simulink model "CACC_4_Robots"  (R2021a)
settings: Solver=FixedStepAuto  StartTime=0.0  StopTime=Tsim  RelTol=1e-3
values from neighbouring files (symbols this model uses):
  h = 1.0    (= 1)    [ros_cacc.m]    (also in ros_cacc2.m)
  k1 = 1    [ros_cacc.m]    (also in ros_cacc2.m)
  k2 = 1    [ros_cacc.m]    (also in ros_cacc2.m)
  r = 1    [ros_cacc.m]    (also in ros_cacc2.m)
  v_0 = 0.5    [ros_cacc.m]    (also in ros_cacc2.m)
  v_threshold = v_thr    (= 0.1)    [ros_cacc.m]    (also in ros_cacc2.m)
undefined symbols (not defined in the file or in its folder): angular, linear
libraries: ros2lib x17, robotcorelib x4
(part 3 of 3)

== system CACC_4_Robots/Subsystem2/controllers/Switch Case Ext. LA/s/Approximation of s around zero ==
  In1 : Inport
  Action Port : ActionPort  ActionPortLabel=if(u1 < 0.01 & u1 > -0.01)
  Taylor approximation 3rd order : Fcn  Expr=0.5*(r+h*u(2))^2*u(1)-0.125*(r+h*u(2))^4*u(1)^3
  Out1 : Outport  VectorParamsAs1DForOutWhenUnconnected=off
  wires:
  In1/1 -> Taylor approximation 3rd order/1
  Taylor approximation 3rd order/1 -> Out1/1

== system CACC_4_Robots/Subsystem2/controllers/Switch Case Ext. LA/s/function s ==
  In1 : Inport
  Action Port : ActionPort  ActionPortLabel=else
  function s : Fcn  Expr=(-1+sqrt(1+u(1)^2*(r+h*u(2))^2))/u(1)
  Out1 : Outport  VectorParamsAs1DForOutWhenUnconnected=off
  wires:
  In1/1 -> function s/1
  function s/1 -> Out1/1

== system CACC_4_Robots/Subsystem/controllers/Switch Case Ext. LA/dz3,dz4 calculation/eq Sig3 line 3/mat ==
  In1 : Inport
  Bus Selector : BusSelector  OutputSignals=curv,v,alpha  OutputAsBus=on
  R11 : Fcn  Expr=u(1)*(r+h*u(2))*sin(u(3))
  R12 : Fcn  Expr=-sin(u(3))
  R21 : Fcn  Expr=sin(u(3))
  R22 : Fcn  Expr=u(1)*(r+h*u(2))*sin(u(3))
  Vector Concatenate6 : Concatenate
  Vector Concatenate7 : Concatenate
  Vector Concatenate8 : Concatenate  Mode=Multidimensional array  ConcatenateDimension=2
  Out1 : Outport  VectorParamsAs1DForOutWhenUnconnected=off
  wires:
  Vector Concatenate8/1 -> Out1/1
  R22/1 -> Vector Concatenate7/2
  R12/1 -> Vector Concatenate7/1
  R21/1 -> Vector Concatenate6/2
  R11/1 -> Vector Concatenate6/1
  Vector Concatenate7/1 -> Vector Concatenate8/2
  Vector Concatenate6/1 -> Vector Concatenate8/1
  Bus Selector/1 -> R12/1, R21/1, R22/1, R11/1
  In1/1 -> Bus Selector/1

== system CACC_4_Robots/Subsystem1/controllers/Switch Case Ext. LA/dz3,dz4 calculation/eq Sig3 line 3/mat ==
  In1 : Inport
  Bus Selector : BusSelector  OutputSignals=curv,v,alpha  OutputAsBus=on
  R11 : Fcn  Expr=u(1)*(r+h*u(2))*sin(u(3))
  R12 : Fcn  Expr=-sin(u(3))
  R21 : Fcn  Expr=sin(u(3))
  R22 : Fcn  Expr=u(1)*(r+h*u(2))*sin(u(3))
  Vector Concatenate6 : Concatenate
  Vector Concatenate7 : Concatenate
  Vector Concatenate8 : Concatenate  Mode=Multidimensional array  ConcatenateDimension=2
  Out1 : Outport  VectorParamsAs1DForOutWhenUnconnected=off
  wires:
  Vector Concatenate8/1 -> Out1/1
  R22/1 -> Vector Concatenate7/2
  R12/1 -> Vector Concatenate7/1
  R21/1 -> Vector Concatenate6/2
  R11/1 -> Vector Concatenate6/1
  Vector Concatenate7/1 -> Vector Concatenate8/2
  Vector Concatenate6/1 -> Vector Concatenate8/1
  Bus Selector/1 -> R12/1, R21/1, R22/1, R11/1
  In1/1 -> Bus Selector/1

== system CACC_4_Robots/Subsystem2/controllers/Switch Case Ext. LA/dz3,dz4 calculation/eq Sig3 line 3/mat ==
  In1 : Inport
  Bus Selector : BusSelector  OutputSignals=curv,v,alpha  OutputAsBus=on
  R11 : Fcn  Expr=u(1)*(r+h*u(2))*sin(u(3))
  R12 : Fcn  Expr=-sin(u(3))
  R21 : Fcn  Expr=sin(u(3))
  R22 : Fcn  Expr=u(1)*(r+h*u(2))*sin(u(3))
  Vector Concatenate6 : Concatenate
  Vector Concatenate7 : Concatenate
  Vector Concatenate8 : Concatenate  Mode=Multidimensional array  ConcatenateDimension=2
  Out1 : Outport  VectorParamsAs1DForOutWhenUnconnected=off
  wires:
  Vector Concatenate8/1 -> Out1/1
  R22/1 -> Vector Concatenate7/2
  R12/1 -> Vector Concatenate7/1
  R21/1 -> Vector Concatenate6/2
  R11/1 -> Vector Concatenate6/1
  Vector Concatenate7/1 -> Vector Concatenate8/2
  Vector Concatenate6/1 -> Vector Concatenate8/1
  Bus Selector/1 -> R12/1, R21/1, R22/1, R11/1
  In1/1 -> Bus Selector/1
